simulink model "rollDynamicsNonLinear"  (R2017a)
settings: Solver=ode3  StartTime=0.0  StopTime=10  FixedStep=0.021  RelTol=1e-3  EnableMultiTasking=on
values from neighbouring files (symbols this model uses):
  armLength = 0.23    [RollDynamics.m]    (also in RollDynamicsPWM-Theta.m; rollDynamics.m)
  enableMisErr = -1    [RollDynamics.m]    (also in RollDynamicsPWM-Theta.m; rollDynamics.m = 1)
  enableOutputPert = -1    [RollDynamics.m]    (also in RollDynamicsPWM-Theta.m)
  enablePwmSaturation = 1    [RollDynamics.m]    (also in RollDynamicsPWM-Theta.m = -1; rollDynamics.m = -1)
  enableRpmSaturation = -1    [RollDynamics.m]    (also in RollDynamicsPWM-Theta.m = 1; rollDynamics.m)
  mode = 1    [RollDynamics.m]    (also in RollDynamicsPWM-Theta.m = -1; rollDynamics.m = -1)
  pwmLowerBound = 1000    [RollDynamics.m]    (also in RollDynamicsPWM-Theta.m = 1100; rollDynamics.m)
  pwmUpperBound = 1800    [RollDynamics.m]    (also in RollDynamicsPWM-Theta.m = 1700; rollDynamics.m)
  rpmLowerBound = 0    [RollDynamics.m]    (also in RollDynamicsPWM-Theta.m; rollDynamics.m)
  rpmUpperBound = 90    [RollDynamics.m]    (also in RollDynamicsPWM-Theta.m; rollDynamics.m)
  Ts = 0.021    [RollDynamics.m]    (also in RollDynamicsPWM-Theta.m; rollDynamics.m)
  Whovering = 1420    [RollDynamics.m]    (also in RollDynamicsPWM-Theta.m = 750; rollDynamics.m)
undefined symbols (not defined in the file or in its folder): motor_den_tf_discrete, motor_num_tf_discrete, roll_den_tf_discrete, roll_num_tf_discrete, sigbuilder_block
libraries: simulink x2
settings Model: Creator=root  LastModifiedBy=userk
settings DataIOCC: LimitDataPoints=on  SaveFormat=Array
settings OptimizationCC: LifeSpan=inf
settings DebuggingCC: SolverPrmCheckMsg=warning  SFUnexpectedBacktrackingDiag=warning  SFNoUnconditionalDefaultTransitionDiag=warning  SFExecutionAtInitializationDiag=none
settings HardwareCC: ProdBitPerPointer=32  ProdBitPerSizeT=32  ProdBitPerPtrDiffT=32  ProdLargestAtomicFloat=None  ProdIntDivRoundTo=Undefined  ProdEndianess=Unspecified  ProdWordSize=32  ProdHWDeviceType=32-bit Generic
settings ModelReferenceCC: PropagateSignalLabelsOutOfModel=off
settings GRTTargetCC: TargetLangStandard=C89/C90 (ANSI)  GeneratePreprocessorConditionals=Disable all
settings ConfigComp: CovMetricSettings=dw  CovHtmlReporting=on  CovSaveCumulativeToWorkspaceVar=on  CovSaveSingleToWorkspaceVar=on  CovExternalEMLEnable=off  CovSFcnEnable=off

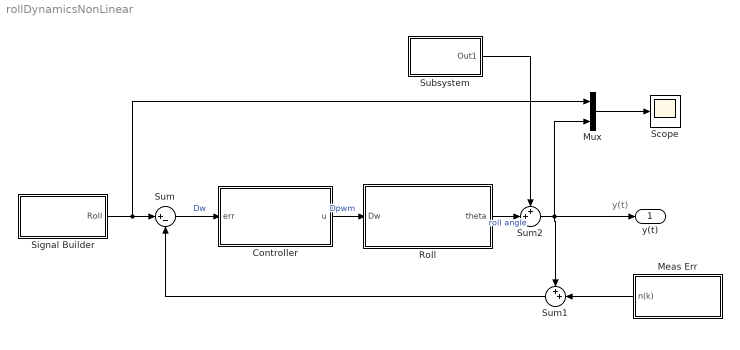
== system rollDynamicsNonLinear ==
  note: y(t)
  "Controller " : Subsystem
  Meas Err : Subsystem
  Mux : Mux  Inputs=2
  "Roll " : Subsystem
  Scope : Scope
  Signal Builder : Subsystem  Tag=STV Subsys  LoadFcn=sigbuilder_block('load');  StartFcn=sigbuilder_block('start');  StopFcn=sigbuilder_block('stop');  ClipboardFcn=sigbuilder_block('clipboard');  mask(Sigbuilder block){tuvar=[0:10]}
      mask help: Simulink:masks:SigbuilderBlock_MD
      mask init:
      | if ~strcmp(get_param(bdroot(gcbh),'SimulationStatus'),'stopped') tuvar = sigbuilder_block('maskInit'); end
      settings: CopyFcn=sigbuilder_block('copy');  DeleteFcn=sigbuilder_block('delete');  ModelCloseFcn=sigbuilder_block('modelClose');  PreSaveFcn=sigbuilder_block('preSave');  PauseFcn=sigbuilder_block('pause');  ContinueFcn=sigbuilder_block('continue');  NameChangeFcn=sigbuilder_block('namechange');  OpenFcn=sigbuilder_block('open',[249.75 0 572.25 465.75 ]);  CloseFcn=sigbuilder_block('close');
      mask Display: plot(0, 0, 100, 100,[2, 2, 32, 32, 2], [68, 8, 8, 68, 68],[32, 2], [38, 38], [32, 19, 2],[53, 60, 44], [32, 17, 17, 2],[16, 16, 31, 31]);txt = getActiveGroup(gcbh);text(2, 100, txt,'verticalAlignment', 'top');
  Subsystem : Subsystem
  Sum : Sum  Inputs=|+-
  Sum1 : Sum  Inputs=++|
  Sum2 : Sum  Inputs=++|
  y(t) : Outport
  wires:
  Signal Builder/1(Roll) -> Mux/1, Sum/1
  Mux/1 -> Scope/1
  Sum/1 -> "Controller "/1("err ")  "Dw"
  "Controller "/1("u ") -> "Roll "/1("Dw ")  "Dpwm"
  Sum1/1 -> Sum/2
  Meas Err/1(n(k)) -> Sum1/2
  "Roll "/1("theta ") -> Sum2/2  "roll angle"
  Sum2/1 -> Sum1/1, Mux/2, y(t)/1
  Subsystem/1(Out1) -> Sum2/1

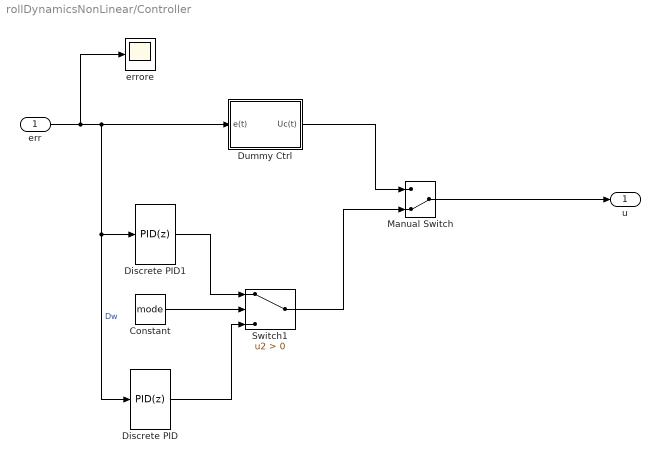
== system rollDynamicsNonLinear/Controller  ==
  "err " : Inport
  Constant : Constant  Value=mode
  Discrete PID : simulink/Continuous/PID Controller  Controller=PID  TimeDomain=Discrete-time  SampleTime=Ts  IntegratorMethod=Forward Euler  FilterMethod=Forward Euler  Form=Parallel  UseFilter=on  ControllerParametersSource=internal  P=-7.49297736675206  I=-7.78960430760415  D=-1.74654639224895  N=78.3475778698318  InitialConditionSource=internal  InitialConditionForIntegrator=0  InitialConditionForFilter=0  ExternalReset=none  LimitOutput=off  UpperSaturationLimit=inf  LowerSaturationLimit=-inf  LinearizeAsGain=off  AntiWindupMode=none  Kb=1  TrackingMode=off  Kt=1  PParamMin=[]  PParamMax=[]  IParamMin=[]  IParamMax=[]  DParamMin=[]  DParamMax=[]  NParamMin=[]  NParamMax=[]  KbParamMin=[]  KbParamMax=[]  KtParamMin=[]  KtParamMax=[]  POutMin=[]  POutMax=[]  IOutMin=[]  IOutMax=[]  DOutMin=[]  DOutMax=[]  NOutMin=[]  NOutMax=[]  KbOutMin=[]  KbOutMax=[]  KtOutMin=[]  KtOutMax=[]  IntegratorOutMin=[]  IntegratorOutMax=[]  FilterOutMin=[]  FilterOutMax=[]  SumOutMin=[]  SumOutMax=[]  SumI1OutMin=[]  SumI1OutMax=[]  SumI2OutMin=[]  SumI2OutMax=[]  SumI3OutMin=[]  SumI3OutMax=[]  SumDOutMin=[]  SumDOutMax=[]  SaturationOutMin=[]  SaturationOutMax=[]  IntegratorContinuousStateAttributes=''  IntegratorStateMustResolveToSignalObject=off  IntegratorRTWStateStorageClass=Auto  FilterContinuousStateAttributes=''  FilterStateMustResolveToSignalObject=off  FilterRTWStateStorageClass=Auto  DifferentiatorICPrevScaledInput=0  DifferentiatorOutMin=[]  DifferentiatorOutMax=[]  InitialConditionSetting=State (most efficient)
  Discrete PID1 : simulink/Continuous/PID Controller  Controller=PID  TimeDomain=Discrete-time  SampleTime=Ts  IntegratorMethod=Forward Euler  FilterMethod=Forward Euler  Form=Parallel  UseFilter=on  ControllerParametersSource=internal  P=-0.00565978055530673  I=-0.539026719553022  D=0  N=100  InitialConditionSource=internal  InitialConditionForIntegrator=0  InitialConditionForFilter=0  ExternalReset=none  LimitOutput=off  UpperSaturationLimit=inf  LowerSaturationLimit=-inf  LinearizeAsGain=off  AntiWindupMode=none  Kb=1  TrackingMode=off  Kt=1  PParamMin=[]  PParamMax=[]  IParamMin=[]  IParamMax=[]  DParamMin=[]  DParamMax=[]  NParamMin=[]  NParamMax=[]  KbParamMin=[]  KbParamMax=[]  KtParamMin=[]  KtParamMax=[]  POutMin=[]  POutMax=[]  IOutMin=[]  IOutMax=[]  DOutMin=[]  DOutMax=[]  NOutMin=[]  NOutMax=[]  KbOutMin=[]  KbOutMax=[]  KtOutMin=[]  KtOutMax=[]  IntegratorOutMin=[]  IntegratorOutMax=[]  FilterOutMin=[]  FilterOutMax=[]  SumOutMin=[]  SumOutMax=[]  SumI1OutMin=[]  SumI1OutMax=[]  SumI2OutMin=[]  SumI2OutMax=[]  SumI3OutMin=[]  SumI3OutMax=[]  SumDOutMin=[]  SumDOutMax=[]  SaturationOutMin=[]  SaturationOutMax=[]  IntegratorContinuousStateAttributes=''  IntegratorStateMustResolveToSignalObject=off  IntegratorRTWStateStorageClass=Auto  FilterContinuousStateAttributes=''  FilterStateMustResolveToSignalObject=off  FilterRTWStateStorageClass=Auto  DifferentiatorICPrevScaledInput=0  DifferentiatorOutMin=[]  DifferentiatorOutMax=[]  InitialConditionSetting=State (most efficient)
  Dummy Ctrl : Subsystem
  Manual Switch : ManualSwitch  CurrentSetting=0
  Switch1 : Switch  Criteria=u2 > Threshold
  errore : Scope
  "u " : Outport
  wires:
  Manual Switch/1 -> "u "/1
  Discrete PID/1 -> Switch1/3
  Dummy Ctrl/1(Uc(t)) -> Manual Switch/1
  Discrete PID1/1 -> Switch1/1
  Constant/1 -> Switch1/2
  Switch1/1 -> Manual Switch/2
  "err "/1 -> errore/1, Discrete PID1/1, Discrete PID/1, Dummy Ctrl/1(e(t))  "Dw"

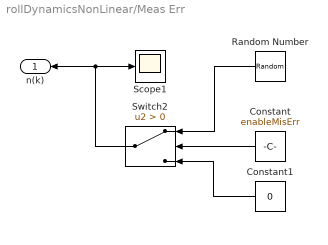
== system rollDynamicsNonLinear/Meas Err ==
  Constant : Constant  Value=enableMisErr
  Constant1 : Constant  Value=0
  Random Number : RandomNumber  Variance=0.5  SampleTime=Ts
  Scope1 : Scope
  Switch2 : Switch  Criteria=u2 > Threshold  SampleTime=Ts
  n(k) : Outport
  wires:
  Constant1/1 -> Switch2/3
  Constant/1 -> Switch2/2
  Random Number/1 -> Switch2/1
  Switch2/1 -> n(k)/1, Scope1/1

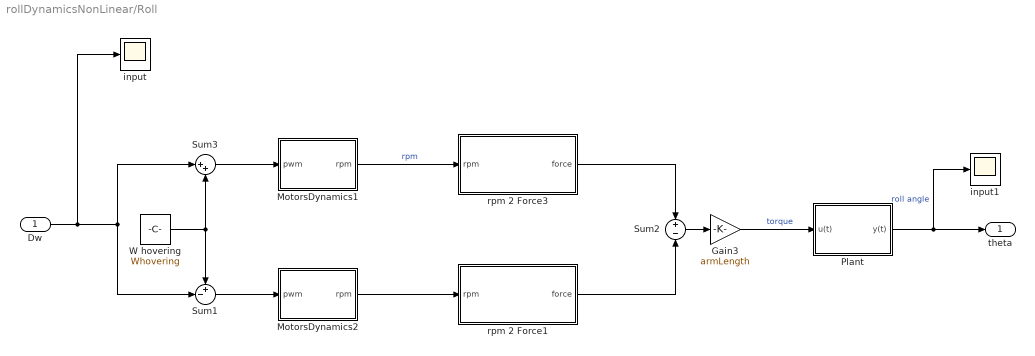
== system rollDynamicsNonLinear/Roll  ==
  "Dw " : Inport
  Gain3 : Gain  Gain=armLength  SampleTime=Ts
  MotorsDynamics1 : Subsystem
  MotorsDynamics2 : Subsystem
  Plant : Subsystem
  Sum1 : Sum  Inputs=+-|
  Sum2 : Sum  Inputs=+|-
  Sum3 : Sum  Inputs=|++
  W hovering : Constant  Value=Whovering  SampleTime=Ts
  input : Scope
  input1 : Scope
  rpm 2 Force1 : Subsystem
  rpm 2 Force3 : Subsystem
  "theta " : Outport
  wires:
  Plant/1(y(t)) -> input1/1, "theta "/1  "roll angle"
  Sum2/1 -> Gain3/1
  W hovering/1 -> Sum3/2, Sum1/1
  Sum1/1 -> MotorsDynamics2/1(pwm)
  MotorsDynamics1/1(rpm) -> rpm 2 Force3/1(rpm)  "rpm"
  MotorsDynamics2/1(rpm) -> rpm 2 Force1/1(rpm)
  Gain3/1 -> Plant/1(u(t))  "torque"
  Sum3/1 -> MotorsDynamics1/1(pwm)
  "Dw "/1 -> input/1, Sum1/2, Sum3/1
  rpm 2 Force3/1(force) -> Sum2/1
  rpm 2 Force1/1(force) -> Sum2/2

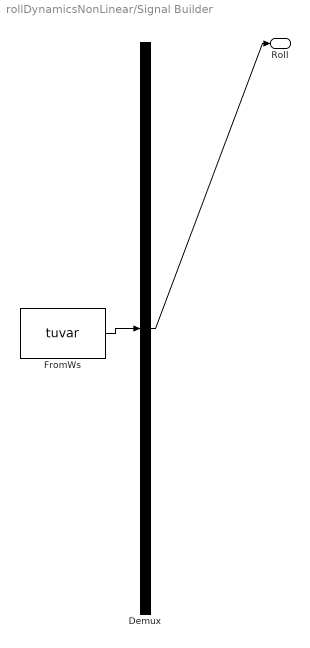
== system rollDynamicsNonLinear/Signal Builder ==
  Demux : Demux  Tag=STV Demux  Outputs=1
  FromWs : FromWorkspace  Tag=STV FromWs  VariableName=tuvar  SampleTime=0
      SigBuilderData=|
      | common.afterFinalStr = 'Extrapolate'
      | common.sampleTime = 0
      | dataSet.timeRange = [0 10]
      | dataSet.name = 'Group 1'
      | sbobj.Groups.Name = 'Group 1'
      | sbobj.Groups.Signals.Name = 'Roll'
      | sbobj.Groups.Signals.XData = [0 4 6 10]
      | sbobj.Groups.Signals.YData = [0 0 0 0]
  Roll : Outport  Tag=STV Outport
  wires:
  FromWs/1 -> Demux/1
  Demux/1 -> Roll/1

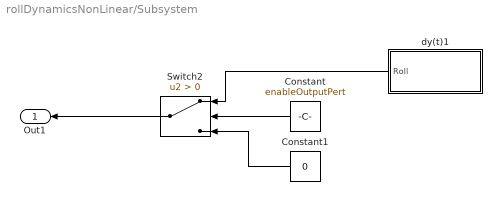
== system rollDynamicsNonLinear/Subsystem ==
  Constant : Constant  Value=enableOutputPert  SampleTime=Ts
  Constant1 : Constant  Value=0
  Switch2 : Switch  Criteria=u2 > Threshold  SampleTime=Ts
  dy(t)1 : Subsystem  Tag=STV Subsys  LoadFcn=sigbuilder_block('load');  StartFcn=sigbuilder_block('start');  StopFcn=sigbuilder_block('stop');  ClipboardFcn=sigbuilder_block('clipboard');  mask(Sigbuilder block){tuvar=[0:10]}
      mask help: Simulink:masks:SigbuilderBlock_MD
      mask init:
      | if ~strcmp(get_param(bdroot(gcbh),'SimulationStatus'),'stopped') tuvar = sigbuilder_block('maskInit'); end
      settings: CopyFcn=sigbuilder_block('copy');  DeleteFcn=sigbuilder_block('delete');  ModelCloseFcn=sigbuilder_block('modelClose');  PreSaveFcn=sigbuilder_block('preSave');  PauseFcn=sigbuilder_block('pause');  ContinueFcn=sigbuilder_block('continue');  NameChangeFcn=sigbuilder_block('namechange');  OpenFcn=sigbuilder_block('open',[234.75 0 602.25 495.75 ]);  CloseFcn=sigbuilder_block('close');
      mask Display: plot(0, 0, 100, 100,[2, 2, 32, 32, 2], [68, 8, 8, 68, 68],[32, 2], [38, 38], [32, 19, 2],[53, 60, 44], [32, 17, 17, 2],[16, 16, 31, 31]);txt = getActiveGroup(gcbh);text(2, 100, txt,'verticalAlignment', 'top');
  Out1 : Outport
  wires:
  Constant1/1 -> Switch2/3
  Constant/1 -> Switch2/2
  Switch2/1 -> Out1/1
  dy(t)1/1(Roll) -> Switch2/1

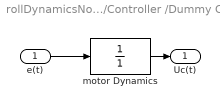
== system rollDynamicsNonLinear/Controller /Dummy Ctrl ==
  e(t) : Inport
  motor Dynamics : DiscreteTransferFcn  Denominator=[1]  SampleTime=Ts
  Uc(t) : Outport
  wires:
  motor Dynamics/1 -> Uc(t)/1
  e(t)/1 -> motor Dynamics/1

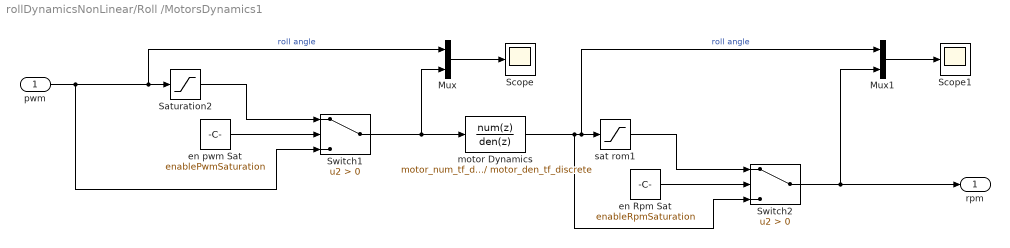
== system rollDynamicsNonLinear/Roll /MotorsDynamics1 ==
  pwm : Inport
  Mux : Mux  Inputs=2
  Mux1 : Mux  Inputs=2
  Saturation2 : Saturate  UpperLimit=pwmUpperBound  LowerLimit=pwmLowerBound  SampleTime=Ts
  Scope : Scope
  Scope1 : Scope
  Switch1 : Switch  Criteria=u2 > Threshold  SampleTime=Ts
  Switch2 : Switch  Criteria=u2 > Threshold  SampleTime=Ts
  en Rpm Sat : Constant  Value=enableRpmSaturation  SampleTime=Ts
  en pwm Sat : Constant  Value=enablePwmSaturation  SampleTime=Ts
  motor Dynamics : DiscreteTransferFcn  Numerator=motor_num_tf_discrete  Denominator=motor_den_tf_discrete  SampleTime=Ts
  sat rom1 : Saturate  UpperLimit=rpmUpperBound  LowerLimit=rpmLowerBound  SampleTime=Ts
  rpm : Outport
  wires:
  en pwm Sat/1 -> Switch1/2
  Switch1/1 -> Mux/2, motor Dynamics/1
  Mux/1 -> Scope/1
  pwm/1 -> Mux/1, Saturation2/1, Switch1/3  "roll angle"
  Saturation2/1 -> Switch1/1
  en Rpm Sat/1 -> Switch2/2
  sat rom1/1 -> Switch2/1
  Switch2/1 -> Mux1/2, rpm/1
  Mux1/1 -> Scope1/1
  motor Dynamics/1 -> Switch2/3, Mux1/1, sat rom1/1  "roll angle"

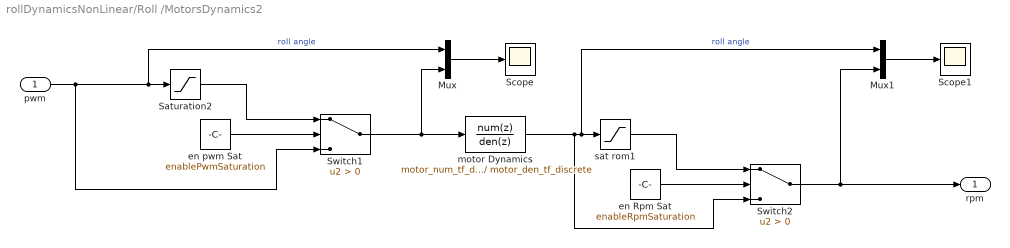
== system rollDynamicsNonLinear/Roll /MotorsDynamics2 ==
  pwm : Inport
  Mux : Mux  Inputs=2
  Mux1 : Mux  Inputs=2
  Saturation2 : Saturate  UpperLimit=pwmUpperBound  LowerLimit=pwmLowerBound  SampleTime=Ts
  Scope : Scope
  Scope1 : Scope
  Switch1 : Switch  Criteria=u2 > Threshold  SampleTime=Ts
  Switch2 : Switch  Criteria=u2 > Threshold  SampleTime=Ts
  en Rpm Sat : Constant  Value=enableRpmSaturation  SampleTime=Ts
  en pwm Sat : Constant  Value=enablePwmSaturation  SampleTime=Ts
  motor Dynamics : DiscreteTransferFcn  Numerator=motor_num_tf_discrete  Denominator=motor_den_tf_discrete  SampleTime=Ts
  sat rom1 : Saturate  UpperLimit=rpmUpperBound  LowerLimit=rpmLowerBound  SampleTime=Ts
  rpm : Outport
  wires:
  en pwm Sat/1 -> Switch1/2
  Switch1/1 -> Mux/2, motor Dynamics/1
  Mux/1 -> Scope/1
  pwm/1 -> Mux/1, Saturation2/1, Switch1/3  "roll angle"
  Saturation2/1 -> Switch1/1
  en Rpm Sat/1 -> Switch2/2
  sat rom1/1 -> Switch2/1
  Switch2/1 -> Mux1/2, rpm/1
  Mux1/1 -> Scope1/1
  motor Dynamics/1 -> Switch2/3, Mux1/1, sat rom1/1  "roll angle"

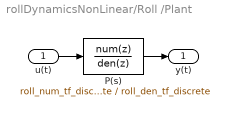
== system rollDynamicsNonLinear/Roll /Plant ==
  u(t) : Inport
  P(s) : DiscreteTransferFcn  Numerator=roll_num_tf_discrete  Denominator=roll_den_tf_discrete  SampleTime=Ts
  y(t) : Outport
  wires:
  P(s)/1 -> y(t)/1
  u(t)/1 -> P(s)/1

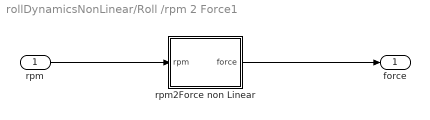
== system rollDynamicsNonLinear/Roll /rpm 2 Force1 ==
  rpm : Inport
  rpm2Force non Linear : MATLAB Function  TreatAsAtomicUnit=on
  force : Outport
  wires:
  rpm2Force non Linear/1(force) -> force/1
  rpm/1 -> rpm2Force non Linear/1(rpm)

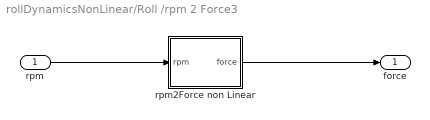
== system rollDynamicsNonLinear/Roll /rpm 2 Force3 ==
  rpm : Inport
  rpm2Force non Linear : MATLAB Function  TreatAsAtomicUnit=on
  force : Outport
  wires:
  rpm/1 -> rpm2Force non Linear/1(rpm)
  rpm2Force non Linear/1(force) -> force/1

== system rollDynamicsNonLinear/Subsystem/dy(t)1 ==
  Demux : Demux  Tag=STV Demux  Outputs=1
  FromWs : FromWorkspace  Tag=STV FromWs  VariableName=tuvar  SampleTime=0
      SigBuilderData=|
      | common.afterFinalStr = 'Extrapolate'
      | common.sampleTime = 0
      | dataSet.timeRange = [0 10]
      | dataSet.name = 'Group 1'
      | sbobj.Groups.Name = 'Group 1'
      | sbobj.Groups.Signals.Name = 'Roll'
      | sbobj.Groups.Signals.XData = [0 4 4 4.06 4.06 10]
      | sbobj.Groups.Signals.YData = [0 0 20 20 0 0]
  Roll : Outport  Tag=STV Outport
  wires:
  Demux/1 -> Roll/1
  FromWs/1 -> Demux/1

== matlab function rollDynamicsNonLinear/Roll /rpm 2 Force1/rpm2Force non Linear ==
  data: rpm input; force output
function force = fcn(rpm)
%#codegen

% Computing Thrust force. It is the result of vertical forces acting on all
% blade elements of one propeller
Radius = 0.115; % m
Radius_in = 9; % in
Ct = 0.18;
rho = 1.225; % kg/m^3
Aprop = pi*Radius^2;

% Convert to RPM
Thrust_newton = Ct*rho*Aprop*(rpm)^2*Radius^2;
Thrust_kg = Thrust_newton/9.81;


force = Thrust_newton;

== matlab function rollDynamicsNonLinear/Roll /rpm 2 Force3/rpm2Force non Linear ==
  data: rpm input; force output
function force = fcn(rpm)
%#codegen

% Computing Thrust force. It is the result of vertical forces acting on all
% blade elements of one propeller
Radius = 0.115; % m
Radius_in = 9; % in
Ct = 0.18;
rho = 1.225; % kg/m^3
Aprop = pi*Radius^2;

% Convert to RPM
Thrust_newton = Ct*rho*Aprop*(rpm)^2*Radius^2;
Thrust_kg = Thrust_newton/9.81;


force = Thrust_newton;
